simulink model "ejercicio_1_05_10_jevg"  (R2021a)
settings: Solver=VariableStepAuto  StartTime=0.0  StopTime=10.0  RelTol=1e-3
libraries: fl_lib x14, nesl_utility x6
settings Model: Creator=luiss  LastModifiedBy=user
settings DebuggingCC: UnconnectedInputMsg=none  UnconnectedOutputMsg=none  UnconnectedLineMsg=none
settings ModelReferenceCC: EnableRefExpFcnMdlSchedulingChecks=off
settings RTWCC: Description=Generic Real-Time Target  DLArmComputeVersion=20.02.1

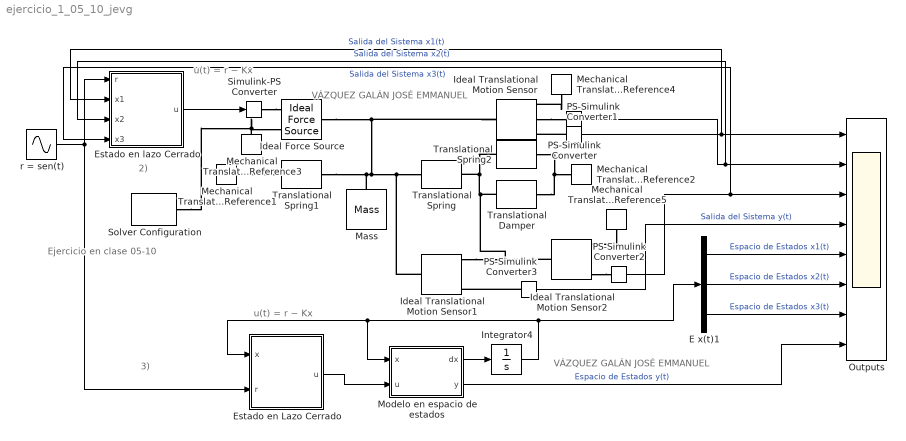
== system ejercicio_1_05_10_jevg ==
  note: u(t) = r − Kx
  note: Ejercicio en clase
      | 05-10
  note: 3)
  note: 2)
  note: VÁZQUEZ GALÁN JOSÉ EMMANUEL
  note: VÁZQUEZ GALÁN JOSÉ EMMANUEL
  note: u(t) = r − Kx
  E x(t)1 : Demux  Outputs=3
  Estado en Lazo Cerrado : MATLAB Function  TreatAsAtomicUnit=on
  Estado en lazo Cerrado : MATLAB Function  TreatAsAtomicUnit=on
  Ideal Force Source : fl_lib/Mechanical/Mechanical Sources/Ideal Force Source
  Ideal Translational Motion Sensor : fl_lib/Mechanical/Mechanical Sensors/Ideal Translational Motion Sensor  offset=0 m
  Ideal Translational Motion Sensor1 : fl_lib/Mechanical/Mechanical Sensors/Ideal Translational Motion Sensor  offset=0 m
  Ideal Translational Motion Sensor2 : fl_lib/Mechanical/Mechanical Sensors/Ideal Translational Motion Sensor  offset=0 m
  Integrator4 : Integrator  InitialCondition=[0;0;0]
  Mass : fl_lib/Mechanical/Translational Elements/Mass  mass=10 kg  num_ports=foundation.enum.numPorts2.one  v_specify=off  v_priority=High  v=0 m/s  v_nominal_specify=off  v_nominal_unit=m/s  v_nominal_value=1  f_specify=off  f_priority=None  f=0 N  f_nominal_specify=off  f_nominal_unit=N  f_nominal_value=1
  Mechanical Translational Reference{1..5} (5 alike) : fl_lib/Mechanical/Translational Elements/Mechanical Translational Reference
  Modelo en espacio de estados : MATLAB Function  TreatAsAtomicUnit=on
  Outputs : Scope  NumInputPorts=8
  PS-Simulink Converter{,1..3} (4 alike) : nesl_utility/PS-Simulink Converter  PhysicalDomain=network_engine_domain  SubClassName=ps_output  LeftPortType=input  RightPortType=output  PseudoPeriodic=off  Frequencies=[]  Unit=inherit  AffineConversion=off
      settings: SourceProductBaseCode=PW,SS
  Simulink-PS Converter : nesl_utility/Simulink-PS Converter  PhysicalDomain=network_engine_domain  SubClassName=ps_input  LeftPortType=input  RightPortType=output  PseudoPeriodic=off  Frequencies=[]  NoiseDistribution=none  NoiseParameters=[]  Unit=1  AffineConversion=off  FilteringAndDerivatives=provide  SimscapeFilterOrder=1  InputFilterTimeConstant=0.001  UdotUserProvided=0
      settings: SourceProductBaseCode=PW,SS
  Solver Configuration : nesl_utility/Solver Configuration  PhysicalDomain=network_engine_domain  SubClassName=solver  LeftPortType=input  RightPortType=generic  Tones=[]  Harmonics=[]  SimulateNoise=off  Profile=off  UseLocalSampling=off  EnableSwitchedLinearOptims=on  FrequencyDomain=off  UseCCode=off  RelTol=0.001  AbsTol=0.001  MinStep=1e-09  ToWorkspace=off  RevertToSquareIcSolve=off  NumHomotopyIterations=100  PhasorMode=off  PhasorModeNumHarmonics=1  DoDC=off  ResidualTolerance=1e-09  UseLocalSolver=off  LocalSolverChoice=NE_BACKWARD_EULER_ADVANCER  LocalSolverSampleTime=0.001  DoFixedCost=off  MaxNonlinIter=3  MaxModeIter=2  ComputeImpulses=off  ImpulseIterations=2  LinearAlgebra=auto  EquationFormulation=NE_TIME_EF  DelaysMemoryBudget=1024  AutomaticFiltering=on  FilteringTimeConstant=0.001  PartitionStorageMethod=AS_NEEDED  PartitionMemoryBudget=1024  PartitionMethod=ROBUST
      settings: SourceProductBaseCode=PW,SS
  Translational Damper : fl_lib/Mechanical/Translational Elements/Translational Damper  D=0.5 N*s/m  v_specify=off  v_priority=None  v=0 m/s  v_nominal_specify=off  v_nominal_unit=m/s  v_nominal_value=1  f_specify=off  f_priority=None  f=0 N  f_nominal_specify=off  f_nominal_unit=N  f_nominal_value=1
  Translational Spring : fl_lib/Mechanical/Translational Elements/Translational Spring  spr_rate=1 N/m  v_specify=off  v_priority=None  v=0 m/s  v_nominal_specify=off  v_nominal_unit=m/s  v_nominal_value=1  f_specify=off  f_priority=None  f=0 N  f_nominal_specify=off  f_nominal_unit=N  f_nominal_value=1  x_specify=off  x_priority=High  x=0 m  x_nominal_specify=off  x_nominal_unit=m  x_nominal_value=1
  Translational Spring1 : fl_lib/Mechanical/Translational Elements/Translational Spring  spr_rate=2 N/m  v_specify=off  v_priority=None  v=0 m/s  v_nominal_specify=off  v_nominal_unit=m/s  v_nominal_value=1  f_specify=off  f_priority=None  f=0 N  f_nominal_specify=off  f_nominal_unit=N  f_nominal_value=1  x_specify=off  x_priority=High  x=0 m  x_nominal_specify=off  x_nominal_unit=m  x_nominal_value=1
  Translational Spring2 : fl_lib/Mechanical/Translational Elements/Translational Spring  spr_rate=0.5 N/m  v_specify=off  v_priority=None  v=0 m/s  v_nominal_specify=off  v_nominal_unit=m/s  v_nominal_value=1  f_specify=off  f_priority=None  f=0 N  f_nominal_specify=off  f_nominal_unit=N  f_nominal_value=1  x_specify=off  x_priority=High  x=0 m  x_nominal_specify=off  x_nominal_unit=m  x_nominal_value=1
  "r = sen(t) " : Sin  SampleTime=0
  wires:
  Integrator4/1 -> Modelo en espacio de estados/1(x), Estado en Lazo Cerrado/1(x), E x(t)1/1
  Modelo en espacio de estados/1(dx) -> Integrator4/1
  Modelo en espacio de estados/2(y) -> Outputs/8  "Espacio de Estados y(t)"
  PS-Simulink Converter3/1 -> Outputs/4  "Salida del Sistema y(t)"
  PS-Simulink Converter2/1 -> Estado en lazo Cerrado/4(x3), Outputs/3  "Salida del Sistema x3(t)"
  PS-Simulink Converter/1 -> Estado en lazo Cerrado/3(x2), Outputs/2  "Salida del Sistema x2(t)"
  PS-Simulink Converter1/1 -> Estado en lazo Cerrado/2(x1), Outputs/1  "Salida del Sistema x1(t)"
  E x(t)1/3 -> Outputs/7  "Espacio de Estados x3(t)"
  E x(t)1/1 -> Outputs/5  "Espacio de Estados x1(t)"
  E x(t)1/2 -> Outputs/6  "Espacio de Estados x2(t)"
  Estado en lazo Cerrado/1(u) -> Simulink-PS Converter/1
  "r = sen(t) "/1 -> Estado en Lazo Cerrado/2(r), Estado en lazo Cerrado/1(r)
  Estado en Lazo Cerrado/1(u) -> Modelo en espacio de estados/2(u)
  connections:
  Translational Spring1/RConn1 -- Ideal Translational Motion Sensor/LConn1 -- Ideal Force Source/LConn1 -- Ideal Translational Motion Sensor1/LConn1 -- Translational Spring/LConn1 -- Mass/LConn1
  Simulink-PS Converter/RConn1 -- Ideal Force Source/RConn1
  Mechanical Translational Reference1/LConn1 -- Translational Spring1/LConn1
  Mechanical Translational Reference3/LConn1 -- Solver Configuration/RConn1 -- Ideal Force Source/RConn2
  Translational Spring2/LConn1 -- Ideal Translational Motion Sensor2/LConn1 -- Ideal Translational Motion Sensor1/RConn1 -- Translational Damper/LConn1 -- Translational Spring/RConn1
  Translational Damper/RConn1 -- Translational Spring2/RConn1 -- Mechanical Translational Reference2/LConn1
  Mechanical Translational Reference4/LConn1 -- Ideal Translational Motion Sensor/RConn1
  Mechanical Translational Reference5/LConn1 -- Ideal Translational Motion Sensor2/RConn1
  PS-Simulink Converter1/LConn1 -- Ideal Translational Motion Sensor/RConn3
  Ideal Translational Motion Sensor/RConn2 -- PS-Simulink Converter/LConn1
  Ideal Translational Motion Sensor2/RConn3 -- PS-Simulink Converter2/LConn1
  PS-Simulink Converter3/LConn1 -- Ideal Translational Motion Sensor1/RConn3

== matlab function ejercicio_1_05_10_jevg/Estado en lazo Cerrado ==
  data: r input; u output; x1 input; x2 input; x3 input
function u = fcn(r,x1,x2,x3)
% Esta función calcula el control u basado en la entrada r y el estado actual del sistema x.

% Definiendo la matriz de ganancias K
K = [137 50 51];

% Organizando las variables de estado en un vector columna
x = [x1,x2,x3]';

% Calculando la señal de control u usando la retroalimentación de estado
u = r - K*x;

== matlab function ejercicio_1_05_10_jevg/Estado en Lazo Cerrado ==
  data: x input; r input; u output
function u = fcn(x,r)
% Esta función calcula el control u basado en la entrada r y el estado actual del sistema x (como vector).

% Definiendo la matriz de ganancias K
K = [137 50 51];

% Calculando la señal de control u usando la retroalimentación de estado
u = r - K*x;

== matlab function ejercicio_1_05_10_jevg/Modelo en espacio de estados ==
  data: x input; dx output; u input; y output
function [dx,y] = fcn(x,u)
% Esta función calcula la derivada del estado dx y la salida y basado en el estado actual x y la señal de control u.

% Definiendo constantes y parámetros del sistema
m1 = 10;
k1 = 2;
k2 = 1;
k3 = 0.5;
b1 = 0.5;

% Definiendo la matriz A del sistema en el espacio de estados
A = [0 1 0; 
    -(k1+k2)/m1 0 k2/m1; 
    k2/b1 0 -(k2+k3)/b1];
% Definiendo la matriz B del sistema en el espacio de estados
B = [0; 
    1/m1; 
    0];

% Definiendo la matriz C para la salida
C=[1 0 -1];

% Calculando la derivada del estado
dx = A*x + B*u;

% Calculando la salida
y = C*x;
